simulink model "force_control_sim2"  (R2013a)
settings: Solver=FixedStepDiscrete  StartTime=0.0  StopTime=5  FixedStep=.001  RelTol=1e-3
undefined symbols (not defined in the file or in its folder): DiscIntNeverNeededParam
libraries: simulink x5
settings Model: Creator=dholley  LastModifiedBy=dholley

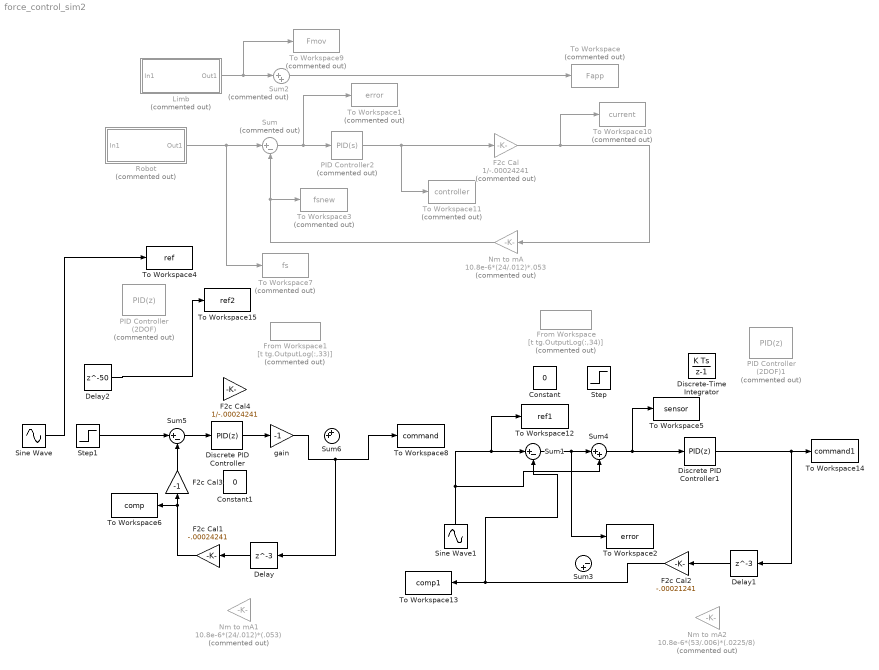
== system force_control_sim2 ==
  Constant : Constant  Value=0
  Constant1 : Constant  Value=0
  Delay : Delay  DelayLength=3  InitialCondition=0  SampleTime=.001
  Delay1 : Delay  DelayLength=3  InitialCondition=0  SampleTime=.001
  Delay2 : Delay  DelayLength=50  InitialCondition=0  SampleTime=.001
  Discrete PID Controller : simulink/Continuous/PID Controller  Controller=PID  TimeDomain=Discrete-time  SampleTime=.001  IntegratorMethod=Forward Euler  FilterMethod=Forward Euler  Form=Parallel  P=-248.280743013811  I=-496561.486027621  D=0  N=100  InitialConditionSource=internal  InitialConditionForIntegrator=0  InitialConditionForFilter=0  ExternalReset=none  LimitOutput=off  UpperSaturationLimit=inf  LowerSaturationLimit=-inf  LinearizeAsGain=off  AntiWindupMode=none  Kb=1  TrackingMode=off  Kt=1  PParamMin=[]  PParamMax=[]  IParamMin=[]  IParamMax=[]  DParamMin=[]  DParamMax=[]  NParamMin=[]  NParamMax=[]  KbParamMin=[]  KbParamMax=[]  KtParamMin=[]  KtParamMax=[]  POutMin=[]  POutMax=[]  IOutMin=[]  IOutMax=[]  DOutMin=[]  DOutMax=[]  NOutMin=[]  NOutMax=[]  KbOutMin=[]  KbOutMax=[]  KtOutMin=[]  KtOutMax=[]  IntegratorOutMin=[]  IntegratorOutMax=[]  FilterOutMin=[]  FilterOutMax=[]  SumOutMin=[]  SumOutMax=[]  SumI1OutMin=[]  SumI1OutMax=[]  SumI2OutMin=[]  SumI2OutMax=[]  SumI3OutMin=[]  SumI3OutMax=[]  SumDOutMin=[]  SumDOutMax=[]  SaturationOutMin=[]  SaturationOutMax=[]  IntegratorContinuousStateAttributes=''  IntegratorStateMustResolveToSignalObject=off  IntegratorRTWStateStorageClass=Auto  FilterContinuousStateAttributes=''  FilterStateMustResolveToSignalObject=off  FilterRTWStateStorageClass=Auto
  Discrete PID Controller1 : simulink/Continuous/PID Controller  Controller=PID  TimeDomain=Discrete-time  SampleTime=.001  IntegratorMethod=Forward Euler  FilterMethod=Forward Euler  Form=Parallel  P=-235.590171722324  I=-471180.343444648  D=0  N=100  InitialConditionSource=internal  InitialConditionForIntegrator=0  InitialConditionForFilter=0  ExternalReset=none  LimitOutput=off  UpperSaturationLimit=inf  LowerSaturationLimit=-inf  LinearizeAsGain=off  AntiWindupMode=none  Kb=1  TrackingMode=off  Kt=1  PParamMin=[]  PParamMax=[]  IParamMin=[]  IParamMax=[]  DParamMin=[]  DParamMax=[]  NParamMin=[]  NParamMax=[]  KbParamMin=[]  KbParamMax=[]  KtParamMin=[]  KtParamMax=[]  POutMin=[]  POutMax=[]  IOutMin=[]  IOutMax=[]  DOutMin=[]  DOutMax=[]  NOutMin=[]  NOutMax=[]  KbOutMin=[]  KbOutMax=[]  KtOutMin=[]  KtOutMax=[]  IntegratorOutMin=[]  IntegratorOutMax=[]  FilterOutMin=[]  FilterOutMax=[]  SumOutMin=[]  SumOutMax=[]  SumI1OutMin=[]  SumI1OutMax=[]  SumI2OutMin=[]  SumI2OutMax=[]  SumI3OutMin=[]  SumI3OutMax=[]  SumDOutMin=[]  SumDOutMax=[]  SaturationOutMin=[]  SaturationOutMax=[]  IntegratorContinuousStateAttributes=''  IntegratorStateMustResolveToSignalObject=off  IntegratorRTWStateStorageClass=Auto  FilterContinuousStateAttributes=''  FilterStateMustResolveToSignalObject=off  FilterRTWStateStorageClass=Auto
  Discrete-Time Integrator : DiscreteIntegrator  SampleTime=.001  ICPrevOutput=DiscIntNeverNeededParam  ICPrevScaledInput=DiscIntNeverNeededParam
  F2c Cal : Gain  Commented=on  Gain=1/-.00024241
  F2c Cal1 : Gain  Gain=-.00024241  SampleTime=.001
  F2c Cal2 : Gain  Gain=-.00021241  SampleTime=.001
  F2c Cal3 : Gain  Gain=-1  SampleTime=.001
  F2c Cal4 : Gain  Gain=1/-.00024241  SampleTime=.001
  From Workspace : FromWorkspace  Commented=on  VariableName=[t tg.OutputLog(:,34)]  SampleTime=0
  From Workspace1 : FromWorkspace  Commented=on  VariableName=[t tg.OutputLog(:,33)]  SampleTime=0
  Limb : Subsystem  Commented=on
  Nm to mA : Gain  Commented=on  Gain=10.8e-6*(24/.012)*.053
  Nm to mA1 : Gain  Commented=on  Gain=10.8e-6*(24/.012)*(.053)  SampleTime=.001
  Nm to mA2 : Gain  Commented=on  Gain=10.8e-6*(53/.006)*(.0225/8)  SampleTime=.001
  PID Controller (2DOF) : simulink/Continuous/PID Controller (2DOF)  Commented=on  Controller=PID  TimeDomain=Discrete-time  SampleTime=.001  IntegratorMethod=Forward Euler  FilterMethod=Forward Euler  Form=Parallel  P=-206.434175056882  I=-412868.350113764  D=0  N=100  b=1  c=1  InitialConditionSource=internal  InitialConditionForIntegrator=0  InitialConditionForFilter=0  ExternalReset=none  LimitOutput=off  UpperSaturationLimit=inf  LowerSaturationLimit=-inf  LinearizeAsGain=on  AntiWindupMode=none  Kb=1  TrackingMode=off  Kt=1  PParamMin=[]  PParamMax=[]  IParamMin=[]  IParamMax=[]  DParamMin=[]  DParamMax=[]  NParamMin=[]  NParamMax=[]  bParamMin=[]  bParamMax=[]  cParamMin=[]  cParamMax=[]  KbParamMin=[]  KbParamMax=[]  KtParamMin=[]  KtParamMax=[]  POutMin=[]  POutMax=[]  IOutMin=[]  IOutMax=[]  DOutMin=[]  DOutMax=[]  NOutMin=[]  NOutMax=[]  bOutMin=[]  bOutMax=[]  cOutMin=[]  cOutMax=[]  KbOutMin=[]  KbOutMax=[]  KtOutMin=[]  KtOutMax=[]  IntegratorOutMin=[]  IntegratorOutMax=[]  FilterOutMin=[]  FilterOutMax=[]  SumOutMin=[]  SumOutMax=[]  Sum1OutMin=[]  Sum1OutMax=[]  Sum2OutMin=[]  Sum2OutMax=[]  Sum3OutMin=[]  Sum3OutMax=[]  SumI1OutMin=[]  SumI1OutMax=[]  SumI2OutMin=[]  SumI2OutMax=[]  SumI3OutMin=[]  SumI3OutMax=[]  SumDOutMin=[]  SumDOutMax=[]  SaturationOutMin=[]  SaturationOutMax=[]  IntegratorContinuousStateAttributes=''  IntegratorStateMustResolveToSignalObject=off  IntegratorRTWStateStorageClass=Auto  FilterContinuousStateAttributes=''  FilterStateMustResolveToSignalObject=off  FilterRTWStateStorageClass=Auto
  PID Controller (2DOF)1 : simulink/Continuous/PID Controller (2DOF)  Commented=on  Controller=PID  TimeDomain=Discrete-time  SampleTime=.001  IntegratorMethod=Forward Euler  FilterMethod=Forward Euler  Form=Parallel  P=-235.590171722324  I=-471180.343444648  D=0  N=100  b=1  c=1  InitialConditionSource=internal  InitialConditionForIntegrator=0  InitialConditionForFilter=0  ExternalReset=none  LimitOutput=off  UpperSaturationLimit=inf  LowerSaturationLimit=-inf  LinearizeAsGain=on  AntiWindupMode=none  Kb=1  TrackingMode=off  Kt=1  PParamMin=[]  PParamMax=[]  IParamMin=[]  IParamMax=[]  DParamMin=[]  DParamMax=[]  NParamMin=[]  NParamMax=[]  bParamMin=[]  bParamMax=[]  cParamMin=[]  cParamMax=[]  KbParamMin=[]  KbParamMax=[]  KtParamMin=[]  KtParamMax=[]  POutMin=[]  POutMax=[]  IOutMin=[]  IOutMax=[]  DOutMin=[]  DOutMax=[]  NOutMin=[]  NOutMax=[]  bOutMin=[]  bOutMax=[]  cOutMin=[]  cOutMax=[]  KbOutMin=[]  KbOutMax=[]  KtOutMin=[]  KtOutMax=[]  IntegratorOutMin=[]  IntegratorOutMax=[]  FilterOutMin=[]  FilterOutMax=[]  SumOutMin=[]  SumOutMax=[]  Sum1OutMin=[]  Sum1OutMax=[]  Sum2OutMin=[]  Sum2OutMax=[]  Sum3OutMin=[]  Sum3OutMax=[]  SumI1OutMin=[]  SumI1OutMax=[]  SumI2OutMin=[]  SumI2OutMax=[]  SumI3OutMin=[]  SumI3OutMax=[]  SumDOutMin=[]  SumDOutMax=[]  SaturationOutMin=[]  SaturationOutMax=[]  IntegratorContinuousStateAttributes=''  IntegratorStateMustResolveToSignalObject=off  IntegratorRTWStateStorageClass=Auto  FilterContinuousStateAttributes=''  FilterStateMustResolveToSignalObject=off  FilterRTWStateStorageClass=Auto
  PID Controller2 : simulink/Continuous/PID Controller  Commented=on  Controller=PID  TimeDomain=Continuous-time  SampleTime=.001  IntegratorMethod=Forward Euler  FilterMethod=Forward Euler  Form=Parallel  P=10  I=500  D=2  N=1  InitialConditionSource=internal  InitialConditionForIntegrator=0  InitialConditionForFilter=0  ExternalReset=none  LimitOutput=off  UpperSaturationLimit=inf  LowerSaturationLimit=-inf  LinearizeAsGain=on  AntiWindupMode=none  Kb=1  TrackingMode=off  Kt=1  PParamMin=[]  PParamMax=[]  IParamMin=[]  IParamMax=[]  DParamMin=[]  DParamMax=[]  NParamMin=[]  NParamMax=[]  KbParamMin=[]  KbParamMax=[]  KtParamMin=[]  KtParamMax=[]  POutMin=[]  POutMax=[]  IOutMin=[]  IOutMax=[]  DOutMin=[]  DOutMax=[]  NOutMin=[]  NOutMax=[]  KbOutMin=[]  KbOutMax=[]  KtOutMin=[]  KtOutMax=[]  IntegratorOutMin=[]  IntegratorOutMax=[]  FilterOutMin=[]  FilterOutMax=[]  SumOutMin=[]  SumOutMax=[]  SumI1OutMin=[]  SumI1OutMax=[]  SumI2OutMin=[]  SumI2OutMax=[]  SumI3OutMin=[]  SumI3OutMax=[]  SumDOutMin=[]  SumDOutMax=[]  SaturationOutMin=[]  SaturationOutMax=[]  IntegratorContinuousStateAttributes=''  IntegratorStateMustResolveToSignalObject=off  IntegratorRTWStateStorageClass=Auto  FilterContinuousStateAttributes=''  FilterStateMustResolveToSignalObject=off  FilterRTWStateStorageClass=Auto
  Robot : Subsystem  Commented=on
  Sine Wave : Sin  Amplitude=.2  Frequency=4*pi  SampleTime=.001
  Sine Wave1 : Sin  Amplitude=.2  Frequency=4*pi  SampleTime=.001
  Step : Step  After=.2  SampleTime=0
  Step1 : Step  After=.2  SampleTime=0
  Sum : Sum  Commented=on  Inputs=|+-
  Sum1 : Sum  Inputs=|+-
  Sum2 : Sum  Commented=on  Inputs=|++
  Sum3 : Sum  Inputs=|+-
  Sum4 : Sum  Inputs=|++
  Sum5 : Sum  Inputs=|+-
  Sum6 : Sum  Inputs=++|
  To Workspace : ToWorkspace  Commented=on  VariableName=Fapp  SampleTime=-1  SaveFormat=Timeseries
  To Workspace1 : ToWorkspace  Commented=on  VariableName=error  SampleTime=-1  SaveFormat=Timeseries
  To Workspace10 : ToWorkspace  Commented=on  VariableName=current  SampleTime=-1  SaveFormat=Timeseries
  To Workspace11 : ToWorkspace  Commented=on  VariableName=controller  SampleTime=-1  SaveFormat=Timeseries
  To Workspace12 : ToWorkspace  VariableName=ref1  SampleTime=.001  SaveFormat=Timeseries
  To Workspace13 : ToWorkspace  VariableName=comp1  SampleTime=.001  SaveFormat=Timeseries
  To Workspace14 : ToWorkspace  VariableName=command1  SampleTime=.001  SaveFormat=Timeseries
  To Workspace15 : ToWorkspace  VariableName=ref2  SampleTime=.001  SaveFormat=Timeseries
  To Workspace2 : ToWorkspace  VariableName=error  SampleTime=.001  SaveFormat=Timeseries
  To Workspace3 : ToWorkspace  Commented=on  VariableName=fsnew  SampleTime=-1  SaveFormat=Timeseries
  To Workspace4 : ToWorkspace  VariableName=ref  SampleTime=.001  SaveFormat=Timeseries
  To Workspace5 : ToWorkspace  VariableName=sensor  SampleTime=.001  SaveFormat=Timeseries
  To Workspace6 : ToWorkspace  VariableName=comp  SampleTime=.001  SaveFormat=Timeseries
  To Workspace7 : ToWorkspace  Commented=on  VariableName=fs  SampleTime=-1  SaveFormat=Timeseries
  To Workspace8 : ToWorkspace  VariableName=command  SampleTime=.001  SaveFormat=Timeseries
  To Workspace9 : ToWorkspace  Commented=on  VariableName=Fmov  SampleTime=-1  SaveFormat=Timeseries
  "gain " : Gain  Gain=-1  SampleTime=.001
  wires:
  Limb/1(Out1) -> To Workspace9/1, Sum2/1
  Sum2/1 -> To Workspace/1
  PID Controller2/1 -> To Workspace11/1, F2c Cal/1
  F2c Cal/1 -> To Workspace10/1, Nm to mA/1
  Nm to mA/1 -> To Workspace3/1, Sum/2
  Sum/1 -> To Workspace1/1, PID Controller2/1
  Robot/1(Out1) -> To Workspace7/1, Sum/1
  Delay1/1 -> F2c Cal2/1
  Delay/1 -> F2c Cal1/1
  F2c Cal1/1 -> F2c Cal3/1, To Workspace6/1
  Discrete PID Controller1/1 -> Delay1/1, To Workspace14/1
  Sine Wave1/1 -> Sum4/2, To Workspace12/1, Sum1/1
  F2c Cal2/1 -> To Workspace13/1, Sum1/2
  Discrete PID Controller/1 -> "gain "/1
  Sum1/1 -> To Workspace2/1, Sum4/1
  Sum4/1 -> To Workspace5/1, Discrete PID Controller1/1
  Sum5/1 -> Discrete PID Controller/1
  F2c Cal3/1 -> Sum5/2
  Delay2/1 -> To Workspace15/1
  "gain "/1 -> Delay/1, To Workspace8/1
  Sine Wave/1 -> To Workspace4/1
  Step1/1 -> Sum5/1

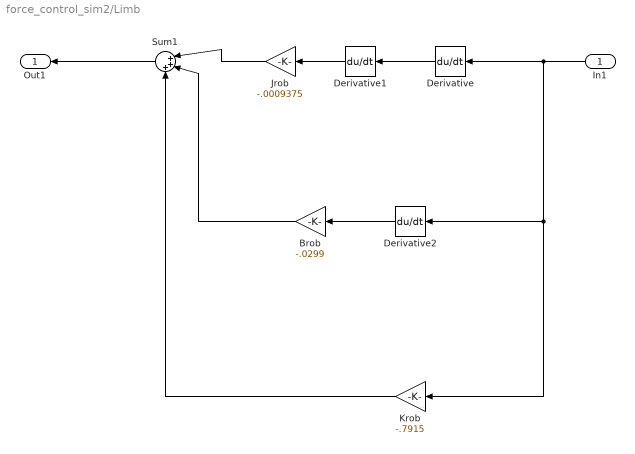
== system force_control_sim2/Limb ==
  In1 : Inport
  Brob : Gain  Gain=-.0299
  Derivative : Derivative
  Derivative1 : Derivative
  Derivative2 : Derivative
  Jrob : Gain  Gain=-.0009375
  Krob : Gain  Gain=-.7915
  Sum1 : Sum  Inputs=|+++
  Out1 : Outport
  wires:
  In1/1 -> Derivative/1, Derivative2/1, Krob/1
  Derivative/1 -> Derivative1/1
  Derivative1/1 -> Jrob/1
  Derivative2/1 -> Brob/1
  Jrob/1 -> Sum1/1
  Brob/1 -> Sum1/2
  Krob/1 -> Sum1/3
  Sum1/1 -> Out1/1

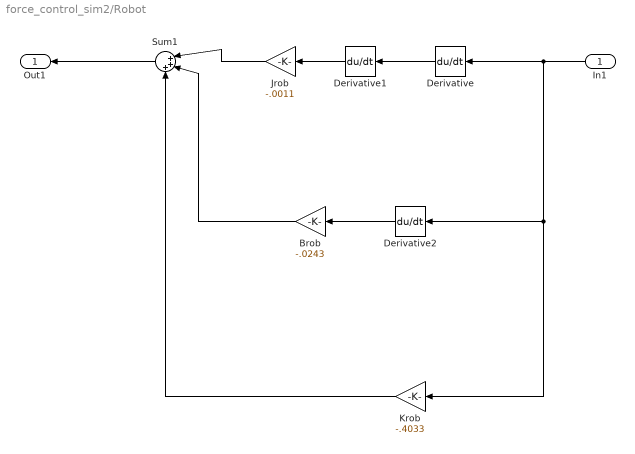
== system force_control_sim2/Robot ==
  In1 : Inport
  Brob : Gain  Gain=-.0243
  Derivative : Derivative
  Derivative1 : Derivative
  Derivative2 : Derivative
  Jrob : Gain  Gain=-.0011
  Krob : Gain  Gain=-.4033
  Sum1 : Sum  Inputs=|+++
  Out1 : Outport
  wires:
  In1/1 -> Derivative/1, Derivative2/1, Krob/1
  Derivative/1 -> Derivative1/1
  Derivative1/1 -> Jrob/1
  Derivative2/1 -> Brob/1
  Jrob/1 -> Sum1/1
  Brob/1 -> Sum1/2
  Krob/1 -> Sum1/3
  Sum1/1 -> Out1/1
